simulink library "NAND"  (R2019b)
settings: Solver=VariableStepAuto  StartTime=0.0  StopTime=10.0  RelTol=1e-3
settings Model: Creator=jthur  LastModifiedBy=JTHURT

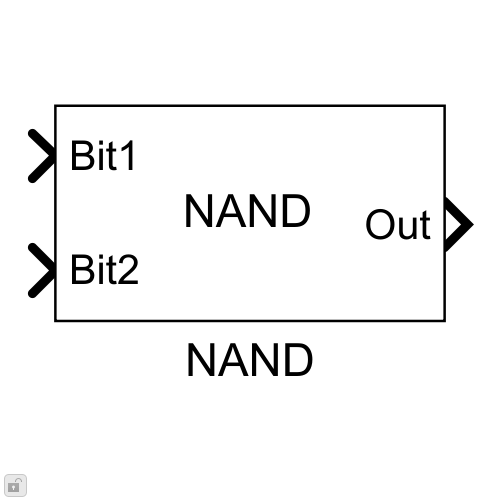
[thumbnail: Simulink's stored preview of the top-level diagram]
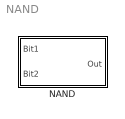
== system NAND ==
  NAND : Subsystem
      mask Display: fprintf("NAND")

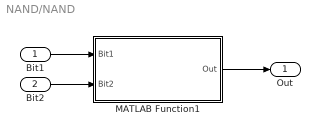
== system NAND/NAND ==
  Bit1 : Inport
  Bit2 : Inport  Port=2
  MATLAB Function1 : MATLAB Function  TreatAsAtomicUnit=on
  Out : Outport
  wires:
  Bit1/1 -> MATLAB Function1/1(Bit1)
  Bit2/1 -> MATLAB Function1/2(Bit2)
  MATLAB Function1/1(Out) -> Out/1

== matlab function NAND/MATLAB Function1 ==
  data: Bit1 input; Out output; Bit2 input
function Out = NAND_Script(Bit1,Bit2)

      
         
if Bit1 && Bit2
    Out = 0;
else
    Out = 1;
end

end
